simulink subsystem "LoadFilter"  (R2024b)
settings: Solver=VariableStepAuto  StartTime=0.0  StopTime=10.0  RelTol=1e-3
undefined symbols (not defined in the file): damp, DT, gmin
libraries: cstblocks x1
settings Model: Creator=jhummel  LastModifiedBy=jhummel
settings ModelReferenceCC: EnableRefExpFcnMdlSchedulingChecks=on
settings RTWCC: GPUComputeCapability=3.5

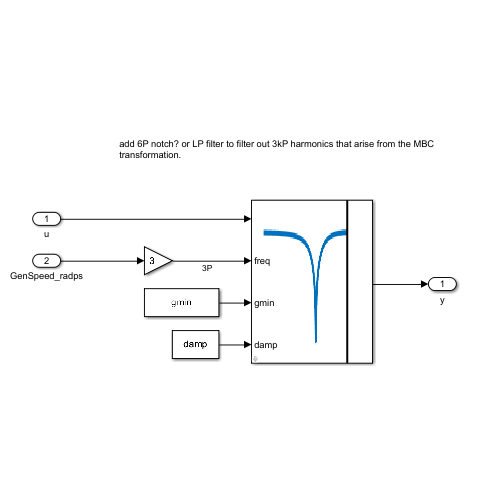
[thumbnail: Simulink's stored preview of the top-level diagram]
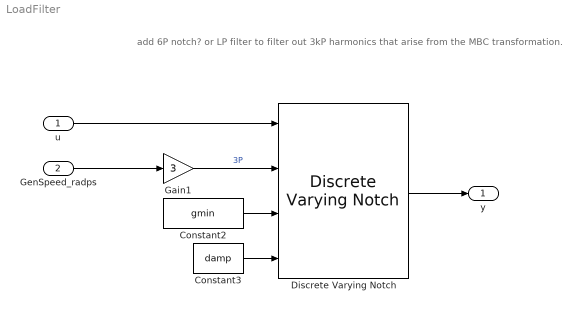
== system LoadFilter ==
  note: add 6P notch? or LP filter to filter out 3kP harmonics that arise from the MBC transformation.
  u : Inport
  GenSpeed_radps : Inport  Port=2
  Constant2 : Constant  Value=gmin
  Constant3 : Constant  Value=damp
  Discrete Varying Notch : cstblocks/Linear Parameter Varying/Discrete Varying Notch  w0=0  Ts=DT
  Gain1 : Gain  Gain=3
  y : Outport
  wires:
  Constant3/1 -> Discrete Varying Notch/4
  u/1 -> Discrete Varying Notch/1
  Gain1/1 -> Discrete Varying Notch/2  "3P"
  GenSpeed_radps/1 -> Gain1/1
  Constant2/1 -> Discrete Varying Notch/3
  Discrete Varying Notch/1 -> y/1
